simulink model "simulacionecuacionbernoullirevisarenverano"  (R2022b)
settings: Solver=VariableStepAuto  StartTime=0.0  StopTime=10.0  RelTol=1e-3
model workspace (MAT data in the model file):
  gradvel = [6 3 5]
settings Model: Creator=gonza  LastModifiedBy=gonza
settings DebuggingCC: AlgebraicLoopMsg=none

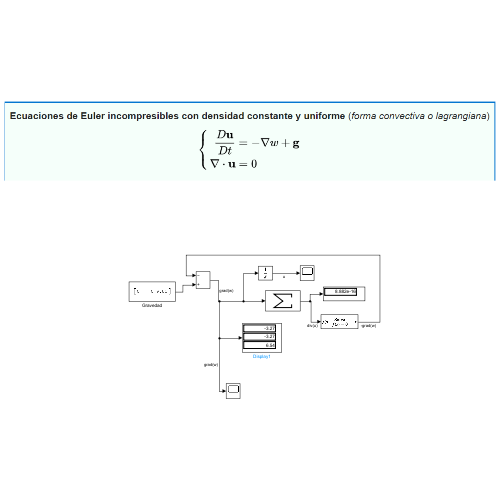
[thumbnail: Simulink's stored preview of the top-level diagram]
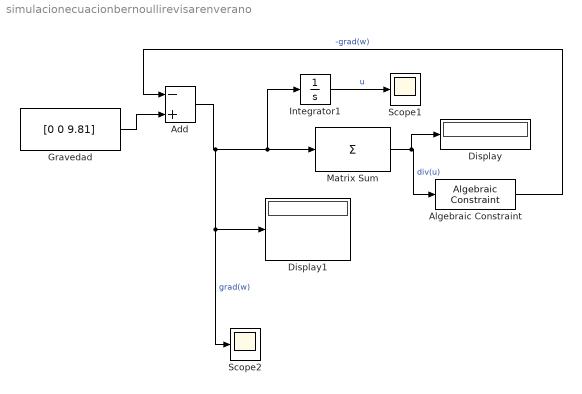
== system simulacionecuacionbernoullirevisarenverano ==
  Add : Sum  Inputs=-+
  Algebraic Constraint : AlgebraicConstraint
  Display : Display
  Display1 : Display
  Gravedad : Constant  Value=[0 0 9.81]
  Integrator1 : Integrator  InitialCondition=[3,2,1]
  Matrix Sum : Sum  Inputs=+
  Scope1 : Scope
  Scope2 : Scope
  wires:
  Gravedad/1 -> Add/2
  Add/1 -> Scope2/1, Display1/1, Integrator1/1, Matrix Sum/1  "grad(w)"
  Matrix Sum/1 -> Display/1, Algebraic Constraint/1  "div(u)"
  Algebraic Constraint/1 -> Add/1  "-grad(w)"
  Integrator1/1 -> Scope1/1  "u"
